simulink library "dlbsBlockMseLoss"  (R2025b)
settings: Solver=VariableStepAuto  StartTime=0.0  StopTime=10.0  RelTol=1e-3
libraries: dlbsBlockAdd x1, dlbsBlockGain x1, dlbsBlockInsertGradientGF x1, dlbsBlockMean x1, dlbsBlockSquare x1
settings Model: Creator=lt6037  LastModifiedBy=lt6037

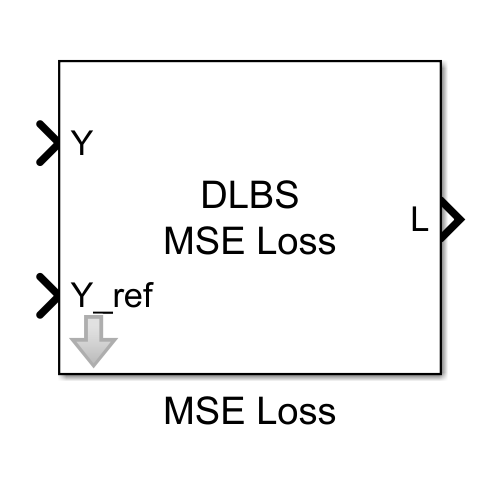
[thumbnail: Simulink's stored preview of the top-level diagram]
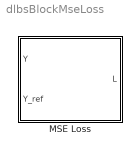
== system dlbsBlockMseLoss ==
  MSE Loss : Subsystem
      mask help: The Mean Squared Error (MSE) Loss block computes the element-wise squared error between a prediction tensor and a reference tensor, and outputs a scalar loss value.
      mask Help: web("dlbsHelpBlockMseLoss.html")
      mask Display: fprintf("DLBS\nMSE Loss")

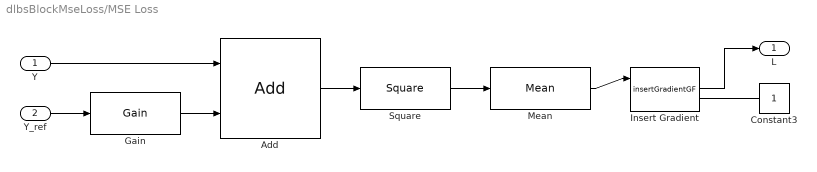
== system dlbsBlockMseLoss/MSE Loss ==
  Y : Inport
  Y_ref : Inport  Port=2
  Add : dlbsBlockAdd/Add  LabelModeActiveChoice=no broadcast  broadcast=off  dims1=1  dims2=1
  Constant3 : Constant
  Gain : dlbsBlockGain/Gain  Gain=-1
  Insert Gradient : dlbsBlockInsertGradientGF/insertGradientGF
  Mean : dlbsBlockMean/Mean
  Square : dlbsBlockSquare/Square
  L : Outport
  wires:
  Constant3/1 -> Insert Gradient/2
  Y_ref/1 -> Gain/1
  Y/1 -> Add/1
  Square/1 -> Mean/1
  Gain/1 -> Add/2
  Add/1 -> Square/1
  Mean/1 -> Insert Gradient/1
  Insert Gradient/1 -> L/1
